simulink model "BD_INSIGHT"  (Simulink 7.9)
settings: Solver=ode1  SolverMode=SingleTasking  StartTime=0.0  StopTime=max(cyc_mph(:,1))  FixedStep=1  MaxStep=1  RelTol=1e-3  AbsTol=1e-3
values from neighbouring files (symbols this model uses):
  ess_on = 1    [insight_data.mat]
  ex_calc = 1    [insight_data.mat]
  fc_emis = 1    [insight_data.mat]
  fc_max_trq = [77.1460442 78.9086076 80.671171 82.2981526 84.060716 85.6876976 87.450261 89.0772426 90.839806 87.1790974 83.382807 79.4509348]    [insight_data.mat]
  fc_trq_scale = 1    [insight_data.mat]
  mc_max_trq = [46.5 46.5 46.5 46.5 46.5 38.2 31.8 27.3 23.9 21.2 19.1 17.4 ... (18 elements, 1x18)]    [insight_data.mat]
  mc_overtrq_factor = 1    [insight_data.mat]
  mc_trq_scale = 1    [insight_data.mat]
  vc_idle_spd = 94    [insight_data.mat]
libraries: lib_transmission x4, lib_wheel x2, lib_controls x2, lib_help x2, lib_accessory x2, lib_outputs x1, lib_interactive x1, lib_drive_cycle x1, lib_energy_storage x1, lib_exhaust x1, lib_fuel_converter x1, lib_electric_machine x1
settings Model: Creator=mokeefe  LastModifiedBy=mokeefe  ExtModeTrigMode=oneshot  ExtModeArmWhenConnect=off
settings Model: ModifiedComment=|
  | mokeefe -- Fri Apr 06 09:18:23 2012 -- Version 1.110
  | Resaving to latest Simulink version.
settings Model: ModifiedHistory=|
  | mokeefe -- Fri Apr 06 09:18:23 2012 -- Version 1.110
  | Resaving to latest Simulink version.
  | 
  | ssprik -- Wed Sep 24 15:00:02 2003 -- Version 1.109
  | 
  | 
  | mokeefe -- Fri Aug 30 07:44:55 2002 -- Version 1.108
  | Changed the input to "mechanical accessory loads <acc>/Mechanical Accessory Loads V2 <acc>" masked parameter input blocks. In R13, the function "not" no longer returns double 1 or double 0 for true and false but instead returns type logical (boolean). Thus, I am now multiplying by double 1 which causes a type conversion to double yielding the desired effect.
  | 
  | 
  | abrooker -- Tue May 14 11:44:46 2002 -- Version 1.107
  | 
  | 
  | mokeefe -- Thu Apr 18 07:58:30 2002 -- Version 1.106
  | saving the model:
  | o "without the model browser open"
  | o with only top-level screen visible
  | o and with "fit to view" enabled
settings DataIOCC: LimitDataPoints=off  SaveOutput=off  SaveTime=off
settings OptimizationCC: BooleanDataType=off
settings DebuggingCC: SaveWithParameterizedLinksMsg=none  SignalResolutionControl=TryResolveAllWithWarning  SolverPrmCheckMsg=none  MultiTaskDSMMsg=warning  MultiTaskCondExecSysMsg=none  UnconnectedLineMsg=none  StrictBusMsg=None
settings HardwareCC: TargetUnknown=on
settings RTWCC: TemplateMakefile=grt_vc.tmf  IncludeERTFirstTime=on
settings GRTTargetCC: CombineOutputUpdateFcns=off  GRTInterface=on

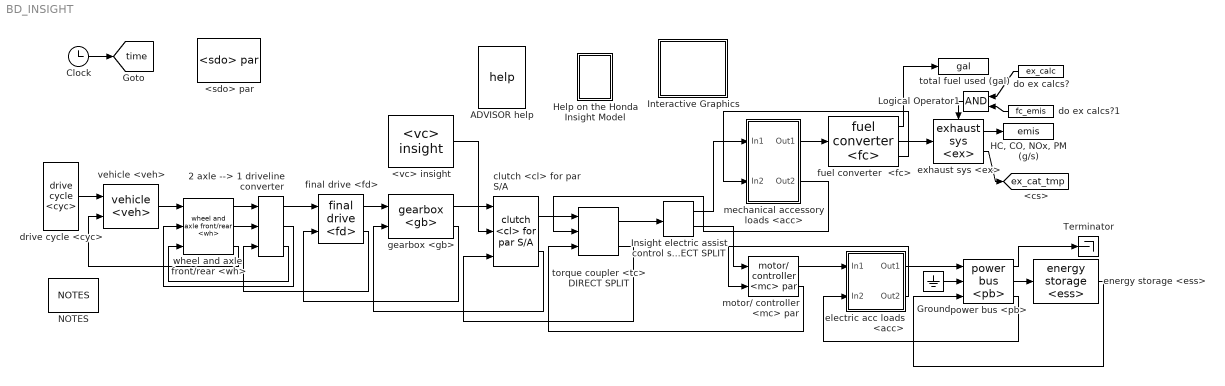
== system BD_INSIGHT ==
  2 axle --> 1 driveline converter : lib_wheel/2 axle --> 1 driveline converter
  <sdo> par : lib_outputs/<sdo> par  SystemSampleTime=-1
  <vc> insight : lib_controls/<vc> insight  SystemSampleTime=-1
      link override config traction control: BlockChoice=traction control 2 axle
  ADVISOR help : lib_help/help  SystemSampleTime=-1
  Clock : Clock
  Ground : Ground
  "HC, CO, NOx, PM (g/s)" : ToWorkspace  VariableName=emis
  Help on the Honda Insight Model : Subsystem
      settings: OpenFcn=web(['file:\\\' which('honda_insight.htm')]);
      mask Display: image(imread('doc_man.jpg'))
  Insight electric assist control strategy <cs> DIRECT SPLIT : lib_controls/Insight electric assist control strategy <cs> DIRECT SPLIT  SystemSampleTime=-1
  Interactive Graphics : Subsystem  BlockChoice=off
      settings: AttributesFormatString=%<BlockChoice>  TemplateBlock=lib_interactive/Interactive Graphics  MemberBlocks=off,on
  Logical Operator1 : Logic
  NOTES : lib_help/NOTES  SystemSampleTime=-1
  Terminator : Terminator
  clutch <cl> for par S/A : lib_transmission/clutch <cl> for par S//A  slip_spd=vc_launch_spd  maxtrq=max(fc_max_trq)*fc_trq_scale+max(mc_max_trq)*mc_overtrq_factor*mc_trq_scale
  do ex calcs? : Constant  Value=ex_calc
  do ex calcs?1 : Constant  Value=fc_emis
  drive cycle <cyc> : lib_drive_cycle/drive cycle <cyc>  SystemSampleTime=-1
  electric acc loads <acc> : Subsystem
      mask Display: image(imread('bdi_acc_elec.bmp'))
  energy storage <ess> : lib_energy_storage/energy storage <ess>  SystemSampleTime=-1
      link override ess config: BlockChoice=energy storage <ess>
  exhaust sys <ex> : lib_exhaust/exhaust sys <ex>  SystemSampleTime=-1
  final drive <fd> : lib_transmission/final drive <fd>  SystemSampleTime=-1
  fuel converter  <fc> : lib_fuel_converter/fuel converter  <fc>  SystemSampleTime=-1
      link override fuel use and EO emis Configurable Subsystem: BlockChoice=fuel use and EO emis
  gearbox <gb> : lib_transmission/gearbox <gb>  SystemSampleTime=-1
  mechanical accessory loads <acc> : Subsystem
      mask Display: image(imread('bdi_acc_pic.bmp'))
  motor/ controller <mc> par : lib_electric_machine/motor// controller <mc> par  SystemSampleTime=-1
  power bus <pb> : lib_power_bus/power bus <pb>  SystemSampleTime=-1
  torque coupler <tc> DIRECT SPLIT : lib_transmission/torque coupler <tc> DIRECT SPLIT  SystemSampleTime=-1
  total fuel used (gal) : ToWorkspace  VariableName=gal
  vehicle <veh> : lib_vehicle/vehicle <veh>  SystemSampleTime=-1
      link override record achieved force outputs/rolling resistance force: BlockChoice=force req'd to overcome rolling resistance (N)
      link override rolling resistance force: BlockChoice=force req'd to overcome rolling resistance (N)
      link override vehicle speed: BlockChoice=vehicle speed (m/s)
  wheel and axle  front/rear <wh> : lib_wheel/wheel and axle  front//rear <wh>  SystemSampleTime=-1
  tag scope: ex_cat_tmp=global, time=global
  wires:
  <vc> insight/1 -> clutch <cl> for par S/A/2
  wheel and axle  front/rear <wh>/3 -> vehicle <veh>/2
  final drive <fd>/2 -> 2 axle --> 1 driveline converter/3
  drive cycle <cyc>/1 -> vehicle <veh>/1
  gearbox <gb>/2 -> final drive <fd>/2
  clutch <cl> for par S/A/2 -> gearbox <gb>/2
  clutch <cl> for par S/A/1 -> torque coupler <tc> DIRECT SPLIT/1
  torque coupler <tc> DIRECT SPLIT/1 -> Insight electric assist control strategy <cs> DIRECT SPLIT/1
  torque coupler <tc> DIRECT SPLIT/2 -> clutch <cl> for par S/A/3
  final drive <fd>/1 -> gearbox <gb>/1
  gearbox <gb>/1 -> clutch <cl> for par S/A/1
  Insight electric assist control strategy <cs> DIRECT SPLIT/2 -> motor/ controller <mc> par/1
  fuel converter  <fc>/2 -> exhaust sys <ex>/1
  do ex calcs?/1 -> Logical Operator1/1
  fuel converter  <fc>/1 -> total fuel used (gal)/1
  exhaust sys <ex>/1 -> "HC, CO, NOx, PM (g/s)"/1
  Logical Operator1/1 -> exhaust sys <ex>/Enable
  do ex calcs?1/1 -> Logical Operator1/2
  motor/ controller <mc> par/2 -> torque coupler <tc> DIRECT SPLIT/3
  Ground/1 -> power bus <pb>/2
  power bus <pb>/2 -> energy storage <ess>/1
  power bus <pb>/1 -> Terminator/1
  energy storage <ess>/1 -> power bus <pb>/3
  exhaust sys <ex>/2 -> [ex_cat_tmp]
  Clock/1 -> [time]
  Insight electric assist control strategy <cs> DIRECT SPLIT/1 -> mechanical accessory loads <acc>/1(In1)
  mechanical accessory loads <acc>/1(Out1) -> fuel converter  <fc>/1
  fuel converter  <fc>/3 -> mechanical accessory loads <acc>/2(In2)
  mechanical accessory loads <acc>/2(Out2) -> torque coupler <tc> DIRECT SPLIT/2
  motor/ controller <mc> par/1 -> electric acc loads <acc>/1(In1)
  electric acc loads <acc>/1(Out1) -> power bus <pb>/1
  power bus <pb>/3 -> electric acc loads <acc>/2(In2)
  electric acc loads <acc>/2(Out2) -> motor/ controller <mc> par/2
  wheel and axle  front/rear <wh>/1 -> 2 axle --> 1 driveline converter/1
  wheel and axle  front/rear <wh>/2 -> 2 axle --> 1 driveline converter/2
  2 axle --> 1 driveline converter/2 -> wheel and axle  front/rear <wh>/2
  2 axle --> 1 driveline converter/3 -> wheel and axle  front/rear <wh>/3
  vehicle <veh>/1 -> wheel and axle  front/rear <wh>/1
  2 axle --> 1 driveline converter/1 -> final drive <fd>/1

== system BD_INSIGHT/Help on the Honda Insight Model ==

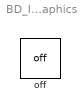
== system BD_INSIGHT/Interactive Graphics ==
  off : lib_interactive/off  Tag=Altia_off  SystemSampleTime=-1

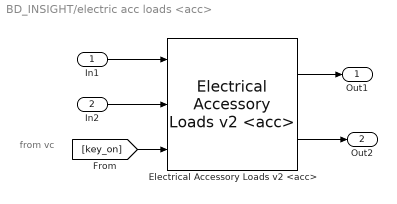
== system BD_INSIGHT/electric acc loads <acc> ==
  note: from vc
  In1 : Inport
  In2 : Inport  Port=2
  Electrical Accessory Loads v2 <acc> : lib_accessory/Electrical Accessory Loads v2 <acc>  load_on=ess_on
      link override backward model/electrical accessories (W): BlockChoice=Electrical Accessories: Time Variable
  Out1 : Outport
  Out2 : Outport  Port=2
  wires:
  In1/1 -> Electrical Accessory Loads v2 <acc>/1
  In2/1 -> Electrical Accessory Loads v2 <acc>/2
  Electrical Accessory Loads v2 <acc>/1 -> Out1/1
  Electrical Accessory Loads v2 <acc>/2 -> Out2/1
  [key_on] -> Electrical Accessory Loads v2 <acc>/3

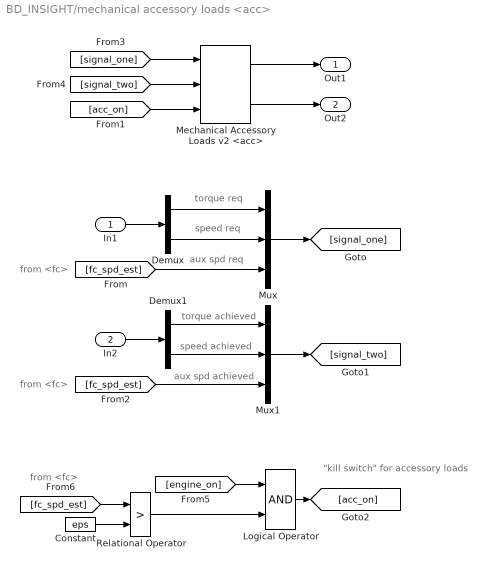
== system BD_INSIGHT/mechanical accessory loads <acc> ==
  note: from <fc>
  note: from <fc>
  note: torque req
  note: speed req
  note: aux spd req
  note: torque achieved
  note: speed achieved
  note: aux spd achieved
  note: from <fc>
  note: "kill switch" for accessory loads
  In1 : Inport
  In2 : Inport  Port=2
  Constant : Constant  Value=eps
  Demux : Demux  Outputs=2
  Demux1 : Demux  Outputs=2
  Logical Operator : Logic
  Mechanical Accessory Loads v2 <acc> : lib_accessory/Mechanical Accessory Loads v2 <acc>  load_on=not(ess_on)*1  acc_max_spd=inf  acc_min_spd=vc_idle_spd+eps  ic_mech_trq=0  ic_mech_pwr=0
      link override backward model/mechanical accessories (Nm): BlockChoice=Mechanical Accessories: Const Mech Var Elect
      link override estimated mechanical torque/mechanical accessories (Nm): BlockChoice=Mechanical Accessories: Const Mech Var Elect
  Mux : Mux  Inputs=3
  Mux1 : Mux  Inputs=3
  Relational Operator : RelationalOperator  Operator=>  InputSameDT=on
  Out1 : Outport
  Out2 : Outport  Port=2
  wires:
  [signal_one] -> Mechanical Accessory Loads v2 <acc>/1
  Mechanical Accessory Loads v2 <acc>/1 -> Out1/1
  Mechanical Accessory Loads v2 <acc>/2 -> Out2/1
  [signal_two] -> Mechanical Accessory Loads v2 <acc>/2
  [acc_on] -> Mechanical Accessory Loads v2 <acc>/3
  Mux/1 -> [signal_one]
  In1/1 -> Demux/1
  Demux/1 -> Mux/1
  Demux/2 -> Mux/2
  [fc_spd_est] -> Mux/3
  Mux1/1 -> [signal_two]
  In2/1 -> Demux1/1
  Demux1/1 -> Mux1/1
  Demux1/2 -> Mux1/2
  [fc_spd_est] -> Mux1/3
  [engine_on] -> Logical Operator/1
  Logical Operator/1 -> [acc_on]
  [fc_spd_est] -> Relational Operator/1
  Constant/1 -> Relational Operator/2
  Relational Operator/1 -> Logical Operator/2
